simulink model "dynamicbalance"  (R2013b)
settings: Solver=ode45  StartTime=0.0  StopTime=10.0  FixedStep=0.0004  RelTol=1e-3
values from neighbouring files (symbols this model uses):
  K = [2*k -1*k;-1*k 2*k]    [q1_assignment.m]    (also in q2.m = [10 -1;-1 10]; q2_assignment.m = [10 -1;-1 10])
  M = [m 0;0 m]    [q1_assignment.m]    (also in q2.m = [2 0;0 8]; q2_assignment.m = [2 0;0 8])
  phi = 2*t*pi    [john (1).m]
  w = sqrt(diag(lam))    [q2.m]
undefined symbols (not defined in the file or in its folder): l, l1, l2, m_b1, m_b2, r_b
settings Model: Creator=Zeerak Nadeem Wyne  LastModifiedBy=Zeerak Nadeem Wyne

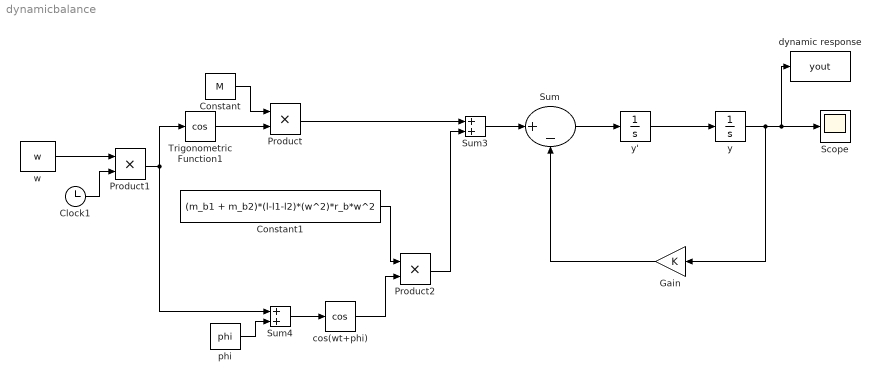
== system dynamicbalance ==
  Clock1 : Clock
  Constant : Constant  Value=M
  Constant1 : Constant  Value=(m_b1 + m_b2)*(l-l1-l2)*(w^2)*r_b*w^2
  Gain : Gain  Gain=K
  Product : Product
  Product1 : Product
  Product2 : Product
  Scope : Scope
  Sum : Sum  Inputs=|+-
  Sum3 : Sum
  Sum4 : Sum
  Trigonometric Function1 : Trigonometry  Operator=cos
  "cos(wt+phi) " : Trigonometry  Operator=cos
  dynamic response : ToWorkspace  VariableName=yout  SampleTime=-1
  "phi " : Constant  Value=phi
  "w " : Constant  Value=w
  "y " : Integrator
  y' : Integrator
  wires:
  Sum3/1 -> Sum/1
  Sum/1 -> y'/1
  y'/1 -> "y "/1
  "y "/1 -> Gain/1, dynamic response/1, Scope/1
  Gain/1 -> Sum/2
  Clock1/1 -> Product1/2
  "w "/1 -> Product1/1
  Trigonometric Function1/1 -> Product/2
  Constant/1 -> Product/1
  Product/1 -> Sum3/1
  "cos(wt+phi) "/1 -> Product2/2
  Constant1/1 -> Product2/1
  Product2/1 -> Sum3/2
  Product1/1 -> Sum4/1, Trigonometric Function1/1
  "phi "/1 -> Sum4/2
  Sum4/1 -> "cos(wt+phi) "/1
